simulink model "tx80211a5s"  (R2015b)
settings: Solver=FixedStepDiscrete  SolverMode=SingleTasking  StartTime=0.0  StopTime=46*tpf  RelTol=1e-3
PreLoadFcn:
  | [stx, stb, spi, spq, ntf, cii, cpp, css] = tx80211a_r0;
InitFcn:
  | if ~exist('srx','var')
  | [stx, stb, spi, spq, ntf, cii, cpp, css] = tx80211a_r0;
  | end
  | bitrate = 6e6; % 6 Mbits per second
  | crf = 2; % constant redundancy factor (from conv enc)
  | nepsc = 16; % #empty+pilot subcarriers
  | ncps = 16; % #cyclic prefix samples
  | ndbpf = 24; % #data bits per frame
  | ncbpf = ndbpf * crf; % #coded bits per frame
  | nscpf = ncbpf + nepsc; % #subcarriers per frame
  | nspf = nscpf + 16; % #samples per frame
  | tps = 1e-6; %tpf/nspf; % sample time
  | tpf = tps*nspf; %ndbpf/bitrate; % frame time
values from neighbouring files (symbols this model uses):
  cpp = [1,1,1,1,-1,-1,-1,1,-1,-1,-1,-1,1,1,-1,1,-1,-1,1,1,-1,1,1,-1,1,1,1,1,1,1,-1,1,     1,1,-1,1,1,-1,-1,1,1,1,-1,1,-1,-1,-1,1,-1,1,-1,-1,1,-1,-1,1,1,1,1,1,-1,-1,1,1,     -1,-1,1,-1,1,-1,1,1,-1,-1,-1,1,1,-1,-1,-1,-1,1,-1,-1,1,-1,1,1,1,1,-1,1,-1,1,-1,1,     -1,-1,-1,-1,-1,1,-1,1,1,-1,1,-1,1,1,1,-1,-1,1,-1,-1,-1,1,1,1,-1,-1,-1,-1,-1,-1,-1]    [tx80211a_r0.m]
  css = repmat(logical([0;1;1;0;1;1;0;0;0;0;0;1;1;0;0;1;1;0;1;0;1;0;0;1;1;1;0;0;1;1;1;1;0;1;1;0;1;0;0;0;0;1;0;1;0;1;0;1;1;1;1;1;0;1;0;0;1;0;1;0;0;0;1;1;0;1;1;1;0;0;0;1;1;1;1;1;1;1;0;0;0;0;1;1;1;0;1;1;1;1;0;0;1;0;1;1;0;0;1;0;0;1;0;0;0;0;0;0;1;0;0;0;1;0;0;1;1;0;0;0;1;0;1;1;1;0;1]),2,1)    [tx80211a_r0.m]
  ntf = nzo+1    [tx80211a_r0.m]
  spi = real(spf)    [tx80211a_r0.m]
  spq = imag(spf)    [tx80211a_r0.m]
  stb = [ssb;szb]    [tx80211a_r0.m]
libraries: simulink x41, hdlsllib x35, dspxfrm3 x1, dspsigops x1, commcnvcod2 x1
(part 1 of 2)
settings Model: Creator=wchen  LastModifiedBy=bdroz
settings SolverCC: PositivePriorityOrder=on
settings DataIOCC: SaveFormat=Array  SaveOutput=off  SignalLogging=off  SaveTime=off
settings OptimizationCC: BlockReduction=off  ConditionallyExecuteInputs=off  DefaultParameterBehavior=Inlined  ExpressionDepthLimit=2147483647  OptimizeModelRefInitCode=on  LifeSpan=1  MaxStackSize=64
settings DebuggingCC: AlgebraicLoopMsg=error  UnderspecifiedInitializationDetection=Classic  MergeDetectMultiDrivingBlocksExec=none  SolverPrmCheckMsg=warning  SingleTaskRateTransMsg=error  ParameterPrecisionLossMsg=none  AllowSymbolicDim=on  StateNameClashWarn=warning
settings HardwareCC: ProdBitPerPointer=32  ProdLargestAtomicFloat=None  ProdIntDivRoundTo=Undefined  ProdEndianess=Unspecified  ProdWordSize=32  ProdHWDeviceType=ASIC/FPGA->ASIC/FPGA  TargetBitPerPointer=64  TargetLongLongMode=on  TargetIntDivRoundTo=Zero  TargetEndianess=LittleEndian  TargetWordSize=64  TargetHWDeviceType=MATLAB Host  ProdEqTarget=off
settings RTWCC: SystemTargetFile=ert.tlc  TemplateMakefile=ert_default_tmf  Description=Embedded Coder  GenerateReport=on  Toolchain=Xilinx Software Development Kit (SDK)  IncludeHyperlinkInReport=on  LaunchReport=on  GenerateTraceInfo=on  GenerateTraceReport=on  GenerateTraceReportSl=on  GenerateTraceReportSf=on  GenerateTraceReportEml=on
settings CodeAppCC: ForceParamTrailComments=on  IgnoreCustomStorageClasses=off  OperatorAnnotations=on  SimulinkDataObjDesc=on  SFDataObjDesc=on  MATLABFcnDesc=on  InsertBlockDesc=on  MATLABSourceComments=on
settings ERTTargetCC: ERTCustomFileTemplate=example_file_process.tlc  ConvertIfToSwitch=on  SuppressUnreachableDefaultCases=on
settings ConfigComp: CovModelRefEnable=Off

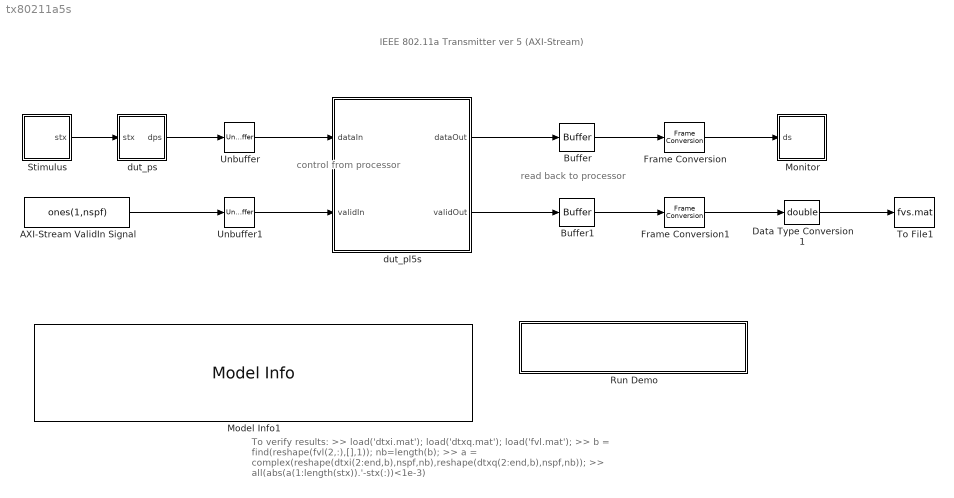
== system tx80211a5s ==
  note: control from
      | processor
  note: IEEE 802.11a Transmitter ver 5 (AXI-Stream)
  note: read back to
      | processor
  note: To verify results:
      | >> load('dtxi.mat'); load('dtxq.mat'); load('fvl.mat');
      | >> b = find(reshape(fvl(2,:),[],1)); nb=length(b);
      | >> a = complex(reshape(dtxi(2:end,b),nspf,nb),reshape(dtxq(2:end,b),nspf,nb));
      | >> all(abs(a(1:length(stx)).'-stx(:))<1e-3)
  AXI-Stream ValidIn Signal : Constant  Value=ones(1,nspf)  OutDataTypeStr=boolean  SampleTime=tpf
  Buffer : Buffer  N=nspf  TreatMby1Signals=One channel  OutputFrames=off
  Buffer1 : Buffer  N=nspf  TreatMby1Signals=One channel  OutputFrames=off
  Data Type Conversion1 : DataTypeConversion  OutDataTypeStr=double
  Frame Conversion : FrameConversion  InheritSamplingMode=off  OutFrame=Sample-based
  Frame Conversion1 : FrameConversion  InheritSamplingMode=off  OutFrame=Sample-based
  Model Info1 : simulink/Model-Wide Utilities/Model Info  Frame=on  DisplayStringWithTags=|  HorizontalTextAlignment=Left  LeftAlignmentValue=0.02  SourceBlockDiagram=tx80211a5s  TagMaxNumber=20
      | This example shows how to use HDL Workflow Advisor to 
      | generate a custom IP core for Zynq SoC evaluation board.
      | 
      | In MATLAB, type the following:
      |   hdladvisor('tx80211a5s/dut_pl5s')
  Monitor : Subsystem
  Run Demo : Subsystem
      settings: OpenFcn=hdladvisor([bdroot, '/led_counter'])
      mask Display: disp('Launch HDL Workflow Advisor')
  Stimulus : Subsystem
  To File1 : ToFile  Filename=fvs.mat  MatrixName=fvs  SampleTime=tpf
  Unbuffer : Unbuffer  SampleBasedProcessing=Same as frame based
  Unbuffer1 : Unbuffer  SampleBasedProcessing=Same as frame based
  dut_pl5s : Subsystem  TreatAsAtomicUnit=on
  dut_ps : Subsystem
  wires:
  Buffer/1 -> Frame Conversion/1
  dut_pl5s/1(dataOut) -> Buffer/1
  Stimulus/1(stx) -> dut_ps/1(stx)
  dut_ps/1(dps) -> Unbuffer/1
  Unbuffer/1 -> dut_pl5s/1(dataIn)
  Frame Conversion/1 -> Monitor/1(ds)
  AXI-Stream ValidIn Signal/1 -> Unbuffer1/1
  Unbuffer1/1 -> dut_pl5s/2(validIn)
  dut_pl5s/2(validOut) -> Buffer1/1
  Buffer1/1 -> Frame Conversion1/1
  Data Type Conversion1/1 -> To File1/1
  Frame Conversion1/1 -> Data Type Conversion1/1

== system tx80211a5s/Monitor ==
  ds : Inport
  Compare To Constant : simulink/Logic and Bit Operations/Compare To Constant  relop=>  const=uint16(0)  OutDataTypeStr=boolean
  Counter Free-Running : simulink/Sources/Counter Free-Running  NumBits=16  tsamp=tpf
  Unpack_int32_into_fix16c1b : Subsystem
  write_srb_to_file : Subsystem
  wires:
  Compare To Constant/1 -> write_srb_to_file/Enable
  Counter Free-Running/1 -> Compare To Constant/1
  ds/1 -> Unpack_int32_into_fix16c1b/1(di32)
  Unpack_int32_into_fix16c1b/2(fvd) -> write_srb_to_file/2(fvl)
  Unpack_int32_into_fix16c1b/1(dts) -> write_srb_to_file/1(srb)

== system tx80211a5s/Run Demo ==

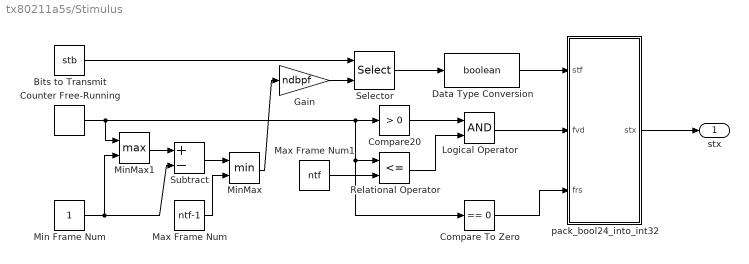
== system tx80211a5s/Stimulus ==
  Bits to Transmit : Constant  Value=stb  SampleTime=tpf
  Compare To Zero : simulink/Logic and Bit Operations/Compare To Zero  relop===  OutDataTypeStr=boolean
  Compare20 : simulink/Logic and Bit Operations/Compare To Zero  relop=>  OutDataTypeStr=boolean
  Counter Free-Running : simulink/Sources/Counter Free-Running  NumBits=16  tsamp=tpf
  Data Type Conversion : DataTypeConversion  OutDataTypeStr=boolean
  Gain : Gain  Gain=ndbpf  OutDataTypeStr=uint16
  Logical Operator : Logic  AllPortsSameDT=off  OutDataTypeStr=boolean
  Max Frame Num : Constant  Value=ntf-1  OutDataTypeStr=uint16  SampleTime=tpf
  Max Frame Num1 : Constant  Value=ntf  OutDataTypeStr=uint16  SampleTime=tpf
  Min Frame Num : Constant  OutDataTypeStr=uint16  SampleTime=tpf
  MinMax : MinMax  Inputs=2  OutDataTypeStr=uint16
  MinMax1 : MinMax  Function=max  Inputs=2
  Relational Operator : RelationalOperator  Operator=<=  OutDataTypeStr=boolean
  Selector : Selector  IndexMode=Zero-based  InputPortWidth=864  IndexOptions=Starting index (port)  Indices=[1 3]  OutputSizes=24
  Subtract : Sum  Inputs=+-  OutDataTypeStr=uint16
  pack_bool24_into_int32 : Subsystem
  stx : Outport
  wires:
  Compare To Zero/1 -> pack_bool24_into_int32/3(frs)
  MinMax1/1 -> Subtract/1
  Subtract/1 -> MinMax/1
  Min Frame Num/1 -> MinMax1/2, Subtract/2
  pack_bool24_into_int32/1(stx) -> stx/1
  Data Type Conversion/1 -> pack_bool24_into_int32/1(stf)
  Selector/1 -> Data Type Conversion/1
  Gain/1 -> Selector/2
  Bits to Transmit/1 -> Selector/1
  MinMax/1 -> Gain/1
  Max Frame Num/1 -> MinMax/2
  Counter Free-Running/1 -> Compare20/1, Relational Operator/1, Compare To Zero/1, MinMax1/1
  Compare20/1 -> Logical Operator/1
  Relational Operator/1 -> Logical Operator/2
  Logical Operator/1 -> pack_bool24_into_int32/2(fvd)
  Max Frame Num1/1 -> Relational Operator/2

== system tx80211a5s/dut_pl5s ==
  dataIn : Inport
  validIn : Inport  Port=2
  PL_dut : Subsystem
  dataOut : Outport  InitialOutput=0
  validOut : Outport  Port=2  InitialOutput=0
  wires:
  dataIn/1 -> PL_dut/1(dps)
  PL_dut/1(dpl) -> dataOut/1
  validIn/1 -> validOut/1, PL_dut/Enable

== system tx80211a5s/dut_ps ==
  stx : Inport
  Logical AND : Logic  IconShape=distinctive  AllPortsSameDT=off  OutDataTypeStr=boolean
  pack_48b_into_int32 : Subsystem
  prepare_frame_ps : Subsystem  TreatAsAtomicUnit=on
  unpack_int32_into_bool24 : Subsystem
  dps : Outport
  wires:
  stx/1 -> unpack_int32_into_bool24/1(di32)
  unpack_int32_into_bool24/3(frs) -> pack_48b_into_int32/3(frs), prepare_frame_ps/2(frs)
  unpack_int32_into_bool24/1(stx) -> prepare_frame_ps/1(stb)
  unpack_int32_into_bool24/2(fvd) -> Logical AND/1, prepare_frame_ps/Enable
  prepare_frame_ps/1(dts) -> pack_48b_into_int32/1(dt48b)
  pack_48b_into_int32/1(dti32) -> dps/1
  Logical AND/1 -> pack_48b_into_int32/2(fvd)
  prepare_frame_ps/2(fvo) -> Logical AND/2

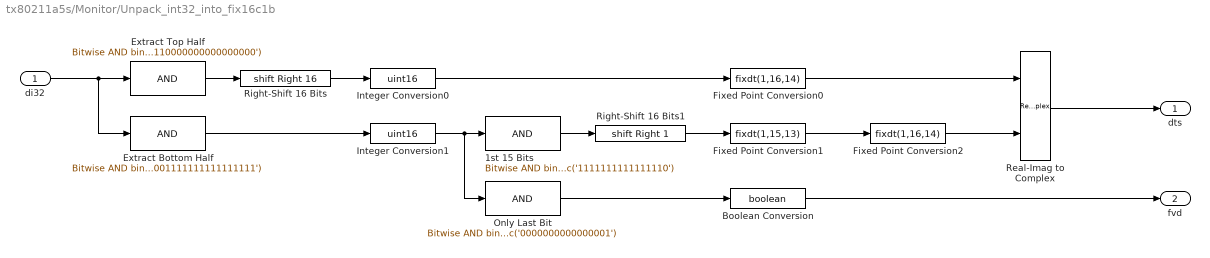
== system tx80211a5s/Monitor/Unpack_int32_into_fix16c1b ==
  di32 : Inport
  1st 15 Bits : simulink/Logic and Bit Operations/Bitwise Operator  logicop=AND  UseBitMask=on  BitMask=bin2dec('1111111111111110')  BitMaskRealWorld=Stored Integer
  Boolean Conversion : DataTypeConversion  OutDataTypeStr=boolean  ConvertRealWorld=Stored Integer (SI)
  Extract Bottom Half : simulink/Logic and Bit Operations/Bitwise Operator  logicop=AND  UseBitMask=on  BitMask=bin2dec('00000000000000001111111111111111')  BitMaskRealWorld=Stored Integer
  Extract Top Half : simulink/Logic and Bit Operations/Bitwise Operator  logicop=AND  UseBitMask=on  BitMask=bin2dec('11111111111111110000000000000000')  BitMaskRealWorld=Stored Integer
  Fixed Point Conversion0 : DataTypeConversion  OutDataTypeStr=fixdt(1,16,14)  ConvertRealWorld=Stored Integer (SI)
      settings: AttributesFormatString=%<OutDataTypeStr>
  Fixed Point Conversion1 : DataTypeConversion  OutDataTypeStr=fixdt(1,15,13)  ConvertRealWorld=Stored Integer (SI)
      settings: AttributesFormatString=%<OutDataTypeStr>
  Fixed Point Conversion2 : DataTypeConversion  OutDataTypeStr=fixdt(1,16,14)
      settings: AttributesFormatString=%<OutDataTypeStr>
  Integer Conversion0 : DataTypeConversion  OutDataTypeStr=uint16  ConvertRealWorld=Stored Integer (SI)
  Integer Conversion1 : DataTypeConversion  OutDataTypeStr=uint16  ConvertRealWorld=Stored Integer (SI)
  Only Last Bit : simulink/Logic and Bit Operations/Bitwise Operator  logicop=AND  UseBitMask=on  BitMask=bin2dec('0000000000000001')  BitMaskRealWorld=Stored Integer
  Real-Imag to Complex : RealImagToComplex
  Right-Shift 16 Bits : ArithShift  BitShiftNumber=16  BitShiftDirection=Right  DiagnosticForOORShift=Error
  Right-Shift 16 Bits1 : ArithShift  BitShiftNumber=1  BitShiftDirection=Right  DiagnosticForOORShift=Error
  dts : Outport
  fvd : Outport  Port=2
  wires:
  Real-Imag to Complex/1 -> dts/1
  Only Last Bit/1 -> Boolean Conversion/1
  Boolean Conversion/1 -> fvd/1
  Fixed Point Conversion0/1 -> Real-Imag to Complex/1
  Fixed Point Conversion2/1 -> Real-Imag to Complex/2
  Extract Bottom Half/1 -> Integer Conversion1/1
  di32/1 -> Extract Bottom Half/1, Extract Top Half/1
  1st 15 Bits/1 -> Right-Shift 16 Bits1/1
  Right-Shift 16 Bits/1 -> Integer Conversion0/1
  Extract Top Half/1 -> Right-Shift 16 Bits/1
  Integer Conversion1/1 -> 1st 15 Bits/1, Only Last Bit/1
  Integer Conversion0/1 -> Fixed Point Conversion0/1
  Fixed Point Conversion1/1 -> Fixed Point Conversion2/1
  Right-Shift 16 Bits1/1 -> Fixed Point Conversion1/1

== system tx80211a5s/Monitor/write_srb_to_file ==
  srb : Inport
  fvl : Inport  Port=2
  Enable : EnablePort
  Complex to Real-Imag : ComplexToRealImag
  Data Type Conversion : DataTypeConversion  OutDataTypeStr=double
  Data Type Conversion1 : DataTypeConversion  OutDataTypeStr=double
  To File : ToFile  Filename=dtxi.mat  MatrixName=dtxi  SampleTime=tpf
  To File1 : ToFile  Filename=fvl.mat  MatrixName=fvl  SampleTime=tpf
  To File2 : ToFile  Filename=dtxq.mat  MatrixName=dtxq  SampleTime=tpf
  wires:
  fvl/1 -> Data Type Conversion1/1
  Data Type Conversion1/1 -> To File1/1
  srb/1 -> Data Type Conversion/1
  Data Type Conversion/1 -> Complex to Real-Imag/1
  Complex to Real-Imag/1 -> To File/1
  Complex to Real-Imag/2 -> To File2/1

== system tx80211a5s/Stimulus/pack_bool24_into_int32 ==
  stf : Inport
  fvd : Inport  Port=2
  frs : Inport  Port=3
  Bit Concat : hdlsllib/HDL Operations/Bit Concat  numInputs=1
  Constant : Constant  Value=false(6,1)  OutDataTypeStr=boolean  SampleTime=tpf
  Vector Concatenate : Concatenate  NumInputs=4
  stx : Outport
  wires:
  Vector Concatenate/1 -> Bit Concat/1
  stf/1 -> Vector Concatenate/1
  fvd/1 -> Vector Concatenate/3
  frs/1 -> Vector Concatenate/4
  Constant/1 -> Vector Concatenate/2
  Bit Concat/1 -> stx/1

== system tx80211a5s/dut_pl5s/PL_dut ==
  dps : Inport
  Enable : EnablePort
  BPSK Modulate : Subsystem  TreatAsAtomicUnit=on
  Interleave : Subsystem  TreatAsAtomicUnit=on
  OFDM Modulate : Subsystem
  Preamble Switch : Subsystem  TreatAsAtomicUnit=on
  Unpack_int32_into_24b : Subsystem
  pack_fpt16c1b_into_int32 : Subsystem
  dpl : Outport  InitialOutput=0
  wires:
  dps/1 -> Unpack_int32_into_24b/1(di32)
  Unpack_int32_into_24b/3(frs) -> Interleave/3(frs), OFDM Modulate/3(frs), Preamble Switch/3(frs)
  OFDM Modulate/2(f8v) -> Preamble Switch/2(f8v)  "f8v"
  pack_fpt16c1b_into_int32/1(dti32) -> dpl/1
  BPSK Modulate/1(s4m) -> OFDM Modulate/1(s4m)
  OFDM Modulate/1(s8s) -> Preamble Switch/1(s8s)
  Preamble Switch/1(s9s) -> pack_fpt16c1b_into_int32/1(dtf16c)
  Preamble Switch/2(f9v) -> pack_fpt16c1b_into_int32/2(fvd)  "f9v"
  BPSK Modulate/2(f4v) -> OFDM Modulate/2(f4v)  "f8v"
  Unpack_int32_into_24b/2(fvd) -> Interleave/2(f3v)  "f8v"
  Unpack_int32_into_24b/1(dts) -> Interleave/1(s2b)
  Interleave/1(s3b) -> BPSK Modulate/1(s3b)
  Interleave/2(f4v) -> BPSK Modulate/2(f3v)

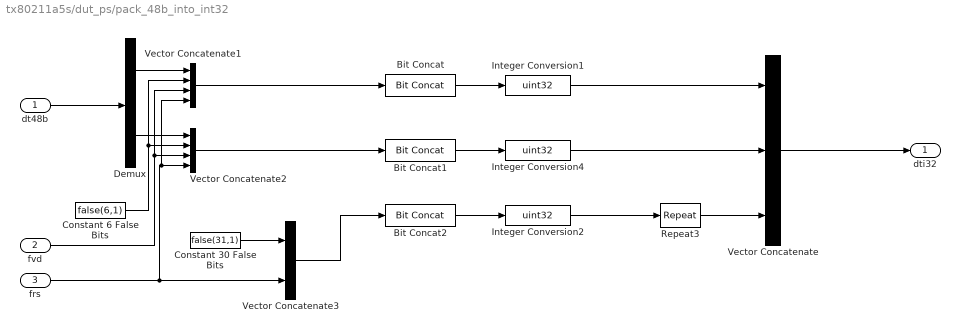
== system tx80211a5s/dut_ps/pack_48b_into_int32 ==
  dt48b : Inport
  fvd : Inport  Port=2
  frs : Inport  Port=3
  Bit Concat : hdlsllib/HDL Operations/Bit Concat  numInputs=1
  Bit Concat1 : hdlsllib/HDL Operations/Bit Concat  numInputs=1
  Bit Concat2 : hdlsllib/HDL Operations/Bit Concat  numInputs=1
  Constant 30 False Bits : Constant  Value=false(31,1)  OutDataTypeStr=boolean  SampleTime=tpf
  Constant 6 False Bits : Constant  Value=false(6,1)  OutDataTypeStr=boolean  SampleTime=tpf
  Demux : Demux  Outputs=2
  Integer Conversion1 : DataTypeConversion  OutDataTypeStr=uint32  ConvertRealWorld=Stored Integer (SI)
  Integer Conversion2 : DataTypeConversion  OutDataTypeStr=uint32  ConvertRealWorld=Stored Integer (SI)
  Integer Conversion4 : DataTypeConversion  OutDataTypeStr=uint32  ConvertRealWorld=Stored Integer (SI)
  Repeat3 : dspsigops/Repeat  N=78  InputProcessing=Columns as channels (frame based)  RateOptions=Enforce single-rate processing  ic=0  mode=Unused parameter value
  Vector Concatenate : Concatenate  NumInputs=3
  Vector Concatenate1 : Concatenate  NumInputs=4
  Vector Concatenate2 : Concatenate  NumInputs=4
  Vector Concatenate3 : Concatenate
  dti32 : Outport
  wires:
  dt48b/1 -> Demux/1
  Vector Concatenate/1 -> dti32/1
  Bit Concat/1 -> Integer Conversion1/1
  Bit Concat1/1 -> Integer Conversion4/1
  Integer Conversion1/1 -> Vector Concatenate/1
  Integer Conversion4/1 -> Vector Concatenate/2
  Demux/1 -> Vector Concatenate1/1
  Demux/2 -> Vector Concatenate2/1
  fvd/1 -> Vector Concatenate1/3, Vector Concatenate2/3
  frs/1 -> Vector Concatenate1/4, Vector Concatenate2/4, Vector Concatenate3/2
  Vector Concatenate1/1 -> Bit Concat/1
  Vector Concatenate2/1 -> Bit Concat1/1
  Constant 6 False Bits/1 -> Vector Concatenate2/2, Vector Concatenate1/2
  Constant 30 False Bits/1 -> Vector Concatenate3/1
  Vector Concatenate3/1 -> Bit Concat2/1
  Bit Concat2/1 -> Integer Conversion2/1
  Integer Conversion2/1 -> Repeat3/1
  Repeat3/1 -> Vector Concatenate/3

== system tx80211a5s/dut_ps/prepare_frame_ps ==
  stb : Inport
  frs : Inport  Port=2
  Enable : EnablePort
  Convolutional Encode : Subsystem  TreatAsAtomicUnit=on
  Scramble : Subsystem  TreatAsAtomicUnit=on
  dts : Outport
  fvo : Outport  Port=2  InitialOutput=0
  wires:
  stb/1 -> Scramble/1(s0b)
  frs/1 -> Scramble/2(frs)
  Scramble/1(s1b) -> Convolutional Encode/1(s1b)
  Scramble/2(f1v) -> Convolutional Encode/2(f1v)
  Convolutional Encode/2(f2v) -> fvo/1
  Convolutional Encode/1(s2b) -> dts/1

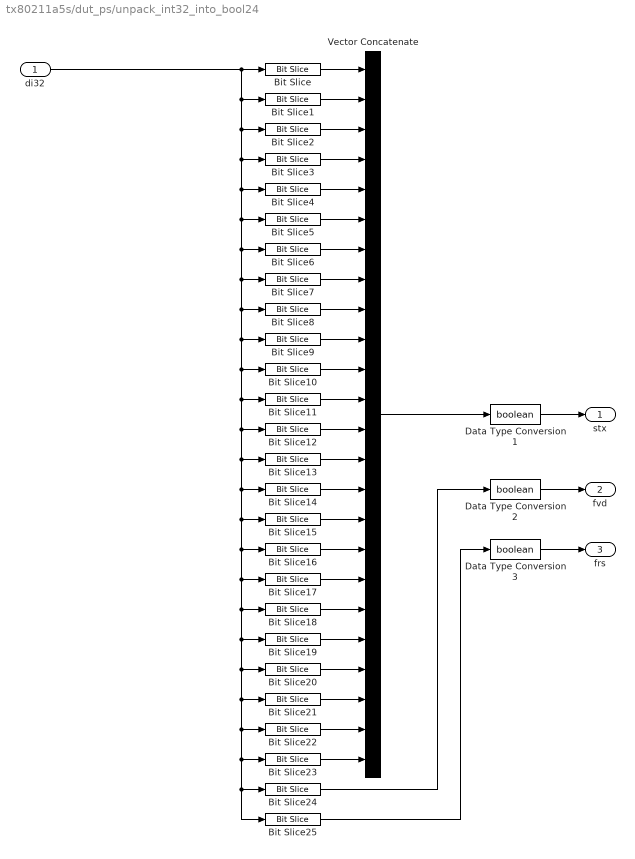
== system tx80211a5s/dut_ps/unpack_int32_into_bool24 ==
  di32 : Inport
  Bit Slice : hdlsllib/HDL Operations/Bit Slice  lidx=31  ridx=31
      settings: AttributesFormatString=%<lidx>
  Bit Slice1 : hdlsllib/HDL Operations/Bit Slice  lidx=30  ridx=30
      settings: AttributesFormatString=%<lidx>
  Bit Slice10 : hdlsllib/HDL Operations/Bit Slice  lidx=21  ridx=21
      settings: AttributesFormatString=%<lidx>
  Bit Slice11 : hdlsllib/HDL Operations/Bit Slice  lidx=20  ridx=20
      settings: AttributesFormatString=%<lidx>
  Bit Slice12 : hdlsllib/HDL Operations/Bit Slice  lidx=19  ridx=19
      settings: AttributesFormatString=%<lidx>
  Bit Slice13 : hdlsllib/HDL Operations/Bit Slice  lidx=18  ridx=18
      settings: AttributesFormatString=%<lidx>
  Bit Slice14 : hdlsllib/HDL Operations/Bit Slice  lidx=17  ridx=17
      settings: AttributesFormatString=%<lidx>
  Bit Slice15 : hdlsllib/HDL Operations/Bit Slice  lidx=16  ridx=16
      settings: AttributesFormatString=%<lidx>
  Bit Slice16 : hdlsllib/HDL Operations/Bit Slice  lidx=15  ridx=15
      settings: AttributesFormatString=%<lidx>
  Bit Slice17 : hdlsllib/HDL Operations/Bit Slice  lidx=14  ridx=14
      settings: AttributesFormatString=%<lidx>
  Bit Slice18 : hdlsllib/HDL Operations/Bit Slice  lidx=13  ridx=13
      settings: AttributesFormatString=%<lidx>
  Bit Slice19 : hdlsllib/HDL Operations/Bit Slice  lidx=12  ridx=12
      settings: AttributesFormatString=%<lidx>
  Bit Slice2 : hdlsllib/HDL Operations/Bit Slice  lidx=29  ridx=29
      settings: AttributesFormatString=%<lidx>
  Bit Slice20 : hdlsllib/HDL Operations/Bit Slice  lidx=11  ridx=11
      settings: AttributesFormatString=%<lidx>
  Bit Slice21 : hdlsllib/HDL Operations/Bit Slice  lidx=10  ridx=10
      settings: AttributesFormatString=%<lidx>
  Bit Slice22 : hdlsllib/HDL Operations/Bit Slice  lidx=9  ridx=9
      settings: AttributesFormatString=%<lidx>
  Bit Slice23 : hdlsllib/HDL Operations/Bit Slice  lidx=8  ridx=8
      settings: AttributesFormatString=%<lidx>
  Bit Slice24 : hdlsllib/HDL Operations/Bit Slice  lidx=1  ridx=1
      settings: AttributesFormatString=%<lidx>
  Bit Slice25 : hdlsllib/HDL Operations/Bit Slice  lidx=0  ridx=0
      settings: AttributesFormatString=%<lidx>
  Bit Slice3 : hdlsllib/HDL Operations/Bit Slice  lidx=28  ridx=28
      settings: AttributesFormatString=%<lidx>
  Bit Slice4 : hdlsllib/HDL Operations/Bit Slice  lidx=27  ridx=27
      settings: AttributesFormatString=%<lidx>
  Bit Slice5 : hdlsllib/HDL Operations/Bit Slice  lidx=26  ridx=26
      settings: AttributesFormatString=%<lidx>
  Bit Slice6 : hdlsllib/HDL Operations/Bit Slice  lidx=25  ridx=25
      settings: AttributesFormatString=%<lidx>
  Bit Slice7 : hdlsllib/HDL Operations/Bit Slice  lidx=24  ridx=24
      settings: AttributesFormatString=%<lidx>
  Bit Slice8 : hdlsllib/HDL Operations/Bit Slice  lidx=23  ridx=23
      settings: AttributesFormatString=%<lidx>
  Bit Slice9 : hdlsllib/HDL Operations/Bit Slice  lidx=22  ridx=22
      settings: AttributesFormatString=%<lidx>
  Data Type Conversion1 : DataTypeConversion  OutDataTypeStr=boolean
  Data Type Conversion2 : DataTypeConversion  OutDataTypeStr=boolean
  Data Type Conversion3 : DataTypeConversion  OutDataTypeStr=boolean
  Vector Concatenate : Concatenate  NumInputs=24
  stx : Outport
  fvd : Outport  Port=2
  frs : Outport  Port=3
  wires:
  Vector Concatenate/1 -> Data Type Conversion1/1
  Bit Slice25/1 -> Data Type Conversion3/1
  Bit Slice24/1 -> Data Type Conversion2/1
  di32/1 -> Bit Slice1/1, Bit Slice2/1, Bit Slice3/1, Bit Slice4/1, Bit Slice5/1, Bit Slice7/1, Bit Slice8/1, Bit Slice9/1, Bit Slice11/1, Bit Slice12/1, Bit Slice13/1, Bit Slice15/1, Bit Slice17/1, Bit Slice18/1, Bit Slice19/1, Bit Slice20/1, Bit Slice21/1, Bit Slice25/1, Bit Slice24/1, Bit Slice23/1, Bit Slice22/1, Bit Slice16/1, Bit Slice14/1, Bit Slice10/1, Bit Slice6/1, Bit Slice/1
  Bit Slice23/1 -> Vector Concatenate/24
  Bit Slice22/1 -> Vector Concatenate/23
  Bit Slice21/1 -> Vector Concatenate/22
  Bit Slice20/1 -> Vector Concatenate/21
  Bit Slice19/1 -> Vector Concatenate/20
  Bit Slice18/1 -> Vector Concatenate/19
  Bit Slice17/1 -> Vector Concatenate/18
  Bit Slice16/1 -> Vector Concatenate/17
  Bit Slice15/1 -> Vector Concatenate/16
  Bit Slice14/1 -> Vector Concatenate/15
  Bit Slice13/1 -> Vector Concatenate/14
  Bit Slice12/1 -> Vector Concatenate/13
  Bit Slice11/1 -> Vector Concatenate/12
  Bit Slice10/1 -> Vector Concatenate/11
  Bit Slice9/1 -> Vector Concatenate/10
  Bit Slice8/1 -> Vector Concatenate/9
  Bit Slice7/1 -> Vector Concatenate/8
  Bit Slice6/1 -> Vector Concatenate/7
  Bit Slice5/1 -> Vector Concatenate/6
  Bit Slice4/1 -> Vector Concatenate/5
  Bit Slice3/1 -> Vector Concatenate/4
  Bit Slice2/1 -> Vector Concatenate/3
  Bit Slice1/1 -> Vector Concatenate/2
  Bit Slice/1 -> Vector Concatenate/1
  Data Type Conversion1/1 -> stx/1
  Data Type Conversion2/1 -> fvd/1
  Data Type Conversion3/1 -> frs/1

== system tx80211a5s/dut_pl5s/PL_dut/BPSK Modulate ==
  s3b : Inport
  f3v : Inport  Port=2
  BPSK Modulate Baseband : Subsystem
  s4m : Outport
  f4v : Outport  Port=2
  wires:
  f3v/1 -> f4v/1
  s3b/1 -> BPSK Modulate Baseband/1(bits)
  BPSK Modulate Baseband/1(symbols) -> s4m/1

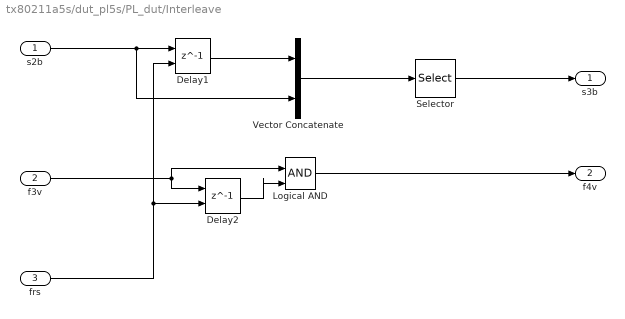
== system tx80211a5s/dut_pl5s/PL_dut/Interleave ==
  s2b : Inport
  f3v : Inport  Port=2
  frs : Inport  Port=3
  Delay1 : Delay  DelayLength=1  ExternalReset=Level  SampleTime=tps
      settings: InputPortMap=u0,r5
  Delay2 : Delay  DelayLength=1  ExternalReset=Level  SampleTime=tps
      settings: InputPortMap=u0,r5
  Logical AND : Logic  IconShape=distinctive  AllPortsSameDT=off  OutDataTypeStr=boolean
  Selector : Selector  IndexMode=Zero-based  InputPortWidth=48  IndexOptions=Index vector (dialog)  Indices=cii  OutputSizes=1
  Vector Concatenate : Concatenate
  s3b : Outport
  f4v : Outport  Port=2
  wires:
  f3v/1 -> Logical AND/1, Delay2/1
  frs/1 -> Delay2/2, Delay1/2
  Delay2/1 -> Logical AND/2
  Logical AND/1 -> f4v/1
  Vector Concatenate/1 -> Selector/1
  Delay1/1 -> Vector Concatenate/1
  s2b/1 -> Vector Concatenate/2, Delay1/1
  Selector/1 -> s3b/1

== system tx80211a5s/dut_pl5s/PL_dut/OFDM Modulate ==
  s4m : Inport
  f4v : Inport  Port=2
  frs : Inport  Port=3
  Frame-Based to Sample-Based : Subsystem
  IFFT HDL Optimized : dspxfrm3/IFFT HDL Optimized  BitReversedOutput=off  Normalize=on  FFTLengthSource=Property  FFTLength=64  RoundingMethod=Floor  OverflowAction=Saturate  ValidInputPort=on  ResetInputPort=on  StartOutputPort=off  EndOutputPort=off  SimulateUsing=Code generation
  Map Symbols to Subcarriers : Subsystem
  Prepend Cyclic Prefix : Subsystem  TreatAsAtomicUnit=on
  s8s : Outport
  f8v : Outport  Port=2
  wires:
  Prepend Cyclic Prefix/1(s8s) -> s8s/1
  Prepend Cyclic Prefix/2(f8v) -> f8v/1  "f8v"
  frs/1 -> Frame-Based to Sample-Based/3(frs), IFFT HDL Optimized/3, Prepend Cyclic Prefix/3(frs), Map Symbols to Subcarriers/3(frs)
  Map Symbols to Subcarriers/2(f5v) -> Frame-Based to Sample-Based/2(f5v)  "f5v"
  s4m/1 -> Map Symbols to Subcarriers/1(s4m)
  f4v/1 -> Map Symbols to Subcarriers/2(f4v)  "f4v"
  Map Symbols to Subcarriers/1(s5m) -> Frame-Based to Sample-Based/1(s5m)
  Frame-Based to Sample-Based/2(f6v) -> IFFT HDL Optimized/2  "f5v"
  Frame-Based to Sample-Based/1(s6m) -> IFFT HDL Optimized/1
  IFFT HDL Optimized/2 -> Prepend Cyclic Prefix/2(f7v)  "f5v"
  IFFT HDL Optimized/1 -> Prepend Cyclic Prefix/1(s7s)

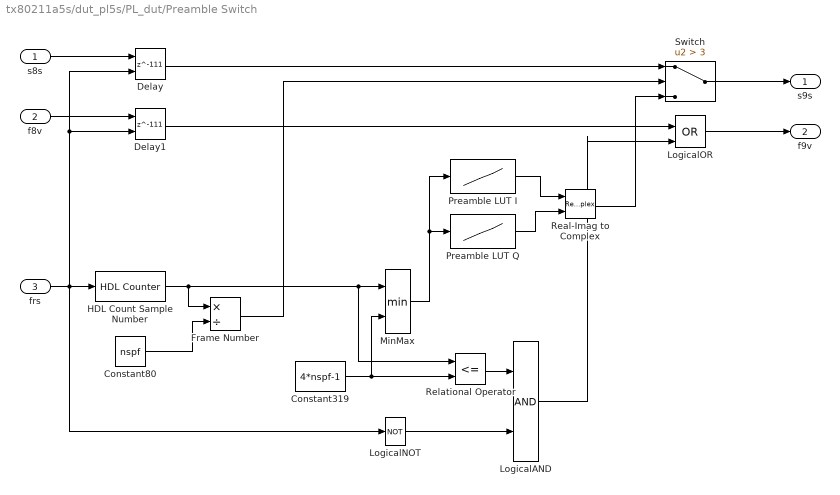
== system tx80211a5s/dut_pl5s/PL_dut/Preamble Switch ==
  s8s : Inport
  f8v : Inport  Port=2
  frs : Inport  Port=3
  Constant319 : Constant  Value=4*nspf-1  OutDataTypeStr=uint16  SampleTime=tps
  Constant80 : Constant  Value=nspf  OutDataTypeStr=uint8  SampleTime=tps
  Delay : Delay  DelayLength=111  ExternalReset=Level  SampleTime=tps
      settings: InputPortMap=u0,r5
  Delay1 : Delay  DelayLength=111  InitialCondition=false  ExternalReset=Level  SampleTime=tps
      settings: InputPortMap=u0,r5
  Frame Number : Product  Inputs=*/  OutDataTypeStr=uint16  SaturateOnIntegerOverflow=on  RndMeth=Zero
  HDL Count Sample Number : hdlsllib/HDL Operations/HDL Counter  CountType=Free running  CountInit=0  CountStep=1  CountMax=3  CountFromType=Initial value  CountFrom=0  CountResetPort=on  CountLoadPort=off  CountEnbPort=off  CountDirPort=off  CountDataType=Unsigned  CountWordLen=16  CountFracLen=0  CountSampTime=1
  LogicalAND : Logic  IconShape=distinctive  AllPortsSameDT=off  OutDataTypeStr=boolean
  LogicalNOT : Logic  Operator=NOT  IconShape=distinctive  AllPortsSameDT=off  OutDataTypeStr=boolean
  LogicalOR : Logic  Operator=OR  IconShape=distinctive  AllPortsSameDT=off  OutDataTypeStr=boolean
  MinMax : MinMax  Inputs=2
  Preamble LUT I : Lookup_n-D  NumberOfTableDimensions=1  BreakpointsForDimension1=[0:1:319]  BreakpointsForDimension1FirstPoint=10  BreakpointsForDimension2FirstPoint=10  BreakpointsForDimension1Spacing=12  BreakpointsForDimension2Spacing=12  IndexSearchMethod=Evenly spaced points  Table=spi  InterpMethod=Flat  DiagnosticForOutOfRangeInput=Error  InternalRulePriority=Speed  OutDataTypeStr=fixdt(1,16,14)  RndMeth=Simplest  InputSameDT=on
  Preamble LUT Q : Lookup_n-D  NumberOfTableDimensions=1  BreakpointsForDimension1=[0:1:319]  BreakpointsForDimension1FirstPoint=10  BreakpointsForDimension2FirstPoint=10  BreakpointsForDimension1Spacing=12  BreakpointsForDimension2Spacing=12  IndexSearchMethod=Evenly spaced points  Table=spq  TableDataTypeStr=fixdt(1,16,14)  InterpMethod=Flat  DiagnosticForOutOfRangeInput=Error  InternalRulePriority=Speed  OutDataTypeStr=fixdt(1,16,14)  RndMeth=Simplest  InputSameDT=on
  Real-Imag to Complex : RealImagToComplex
  Relational Operator : RelationalOperator  Operator=<=  OutDataTypeStr=boolean
  Switch : Switch  Criteria=u2 > Threshold  Threshold=3
  s9s : Outport
  f9v : Outport  Port=2
  wires:
  f8v/1 -> Delay1/1
  frs/1 -> Delay/2, Delay1/2, LogicalNOT/1, HDL Count Sample Number/1
  Switch/1 -> s9s/1
  s8s/1 -> Delay/1
  Real-Imag to Complex/1 -> Switch/3
  Constant80/1 -> Frame Number/2
  Delay/1 -> Switch/1
  Frame Number/1 -> Switch/2
  HDL Count Sample Number/1 -> Relational Operator/1, MinMax/1, Frame Number/1
  Constant319/1 -> MinMax/2, Relational Operator/2
  MinMax/1 -> Preamble LUT Q/1, Preamble LUT I/1
  LogicalOR/1 -> f9v/1
  LogicalNOT/1 -> LogicalAND/2
  Relational Operator/1 -> LogicalAND/1
  LogicalAND/1 -> LogicalOR/2
  Delay1/1 -> LogicalOR/1
  Preamble LUT I/1 -> Real-Imag to Complex/1
  Preamble LUT Q/1 -> Real-Imag to Complex/2

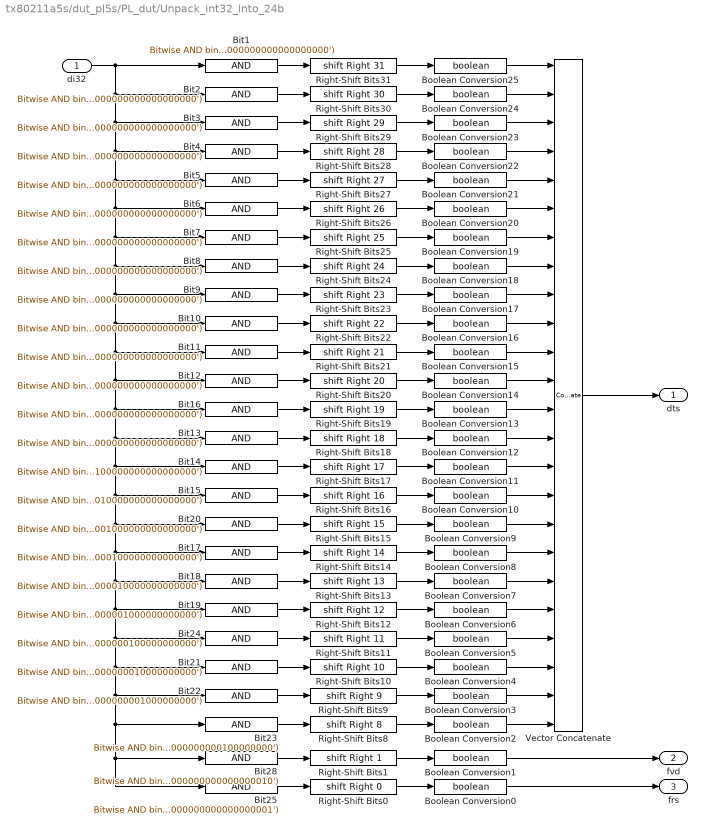
== system tx80211a5s/dut_pl5s/PL_dut/Unpack_int32_into_24b ==
  di32 : Inport
  Bit1 : simulink/Logic and Bit Operations/Bitwise Operator  logicop=AND  UseBitMask=on  BitMask=bin2dec('10000000000000000000000000000000')  BitMaskRealWorld=Stored Integer
      settings: AttributesFormatString=%<logicop>%<BitMask>
  Bit10 : simulink/Logic and Bit Operations/Bitwise Operator  logicop=AND  UseBitMask=on  BitMask=bin2dec('00000000010000000000000000000000')  BitMaskRealWorld=Stored Integer
      settings: AttributesFormatString=%<logicop>%<BitMask>
  Bit11 : simulink/Logic and Bit Operations/Bitwise Operator  logicop=AND  UseBitMask=on  BitMask=bin2dec('00000000001000000000000000000000')  BitMaskRealWorld=Stored Integer
      settings: AttributesFormatString=%<logicop>%<BitMask>
  Bit12 : simulink/Logic and Bit Operations/Bitwise Operator  logicop=AND  UseBitMask=on  BitMask=bin2dec('00000000000100000000000000000000')  BitMaskRealWorld=Stored Integer
      settings: AttributesFormatString=%<logicop>%<BitMask>
  Bit13 : simulink/Logic and Bit Operations/Bitwise Operator  logicop=AND  UseBitMask=on  BitMask=bin2dec('00000000000001000000000000000000')  BitMaskRealWorld=Stored Integer
      settings: AttributesFormatString=%<logicop>%<BitMask>
  Bit14 : simulink/Logic and Bit Operations/Bitwise Operator  logicop=AND  UseBitMask=on  BitMask=bin2dec('00000000000000100000000000000000')  BitMaskRealWorld=Stored Integer
      settings: AttributesFormatString=%<logicop>%<BitMask>
  Bit15 : simulink/Logic and Bit Operations/Bitwise Operator  logicop=AND  UseBitMask=on  BitMask=bin2dec('00000000000000010000000000000000')  BitMaskRealWorld=Stored Integer
      settings: AttributesFormatString=%<logicop>%<BitMask>
  Bit16 : simulink/Logic and Bit Operations/Bitwise Operator  logicop=AND  UseBitMask=on  BitMask=bin2dec('00000000000010000000000000000000')  BitMaskRealWorld=Stored Integer
      settings: AttributesFormatString=%<logicop>%<BitMask>
  Bit17 : simulink/Logic and Bit Operations/Bitwise Operator  logicop=AND  UseBitMask=on  BitMask=bin2dec('00000000000000000100000000000000')  BitMaskRealWorld=Stored Integer
      settings: AttributesFormatString=%<logicop>%<BitMask>
  Bit18 : simulink/Logic and Bit Operations/Bitwise Operator  logicop=AND  UseBitMask=on  BitMask=bin2dec('00000000000000000010000000000000')  BitMaskRealWorld=Stored Integer
      settings: AttributesFormatString=%<logicop>%<BitMask>
  Bit19 : simulink/Logic and Bit Operations/Bitwise Operator  logicop=AND  UseBitMask=on  BitMask=bin2dec('00000000000000000001000000000000')  BitMaskRealWorld=Stored Integer
      settings: AttributesFormatString=%<logicop>%<BitMask>
  Bit2 : simulink/Logic and Bit Operations/Bitwise Operator  logicop=AND  UseBitMask=on  BitMask=bin2dec('01000000000000000000000000000000')  BitMaskRealWorld=Stored Integer
      settings: AttributesFormatString=%<logicop>%<BitMask>
  Bit20 : simulink/Logic and Bit Operations/Bitwise Operator  logicop=AND  UseBitMask=on  BitMask=bin2dec('00000000000000001000000000000000')  BitMaskRealWorld=Stored Integer
      settings: AttributesFormatString=%<logicop>%<BitMask>
  Bit21 : simulink/Logic and Bit Operations/Bitwise Operator  logicop=AND  UseBitMask=on  BitMask=bin2dec('00000000000000000000010000000000')  BitMaskRealWorld=Stored Integer
      settings: AttributesFormatString=%<logicop>%<BitMask>
  Bit22 : simulink/Logic and Bit Operations/Bitwise Operator  logicop=AND  UseBitMask=on  BitMask=bin2dec('00000000000000000000001000000000')  BitMaskRealWorld=Stored Integer
      settings: AttributesFormatString=%<logicop>%<BitMask>
  Bit23 : simulink/Logic and Bit Operations/Bitwise Operator  logicop=AND  UseBitMask=on  BitMask=bin2dec('00000000000000000000000100000000')  BitMaskRealWorld=Stored Integer
      settings: AttributesFormatString=%<logicop>%<BitMask>
  Bit24 : simulink/Logic and Bit Operations/Bitwise Operator  logicop=AND  UseBitMask=on  BitMask=bin2dec('00000000000000000000100000000000')  BitMaskRealWorld=Stored Integer
      settings: AttributesFormatString=%<logicop>%<BitMask>
  Bit25 : simulink/Logic and Bit Operations/Bitwise Operator  logicop=AND  UseBitMask=on  BitMask=bin2dec('00000000000000000000000000000001')  BitMaskRealWorld=Stored Integer
      settings: AttributesFormatString=%<logicop>%<BitMask>
  Bit28 : simulink/Logic and Bit Operations/Bitwise Operator  logicop=AND  UseBitMask=on  BitMask=bin2dec('00000000000000000000000000000010')  BitMaskRealWorld=Stored Integer
      settings: AttributesFormatString=%<logicop>%<BitMask>
  Bit3 : simulink/Logic and Bit Operations/Bitwise Operator  logicop=AND  UseBitMask=on  BitMask=bin2dec('00100000000000000000000000000000')  BitMaskRealWorld=Stored Integer
      settings: AttributesFormatString=%<logicop>%<BitMask>
  Bit4 : simulink/Logic and Bit Operations/Bitwise Operator  logicop=AND  UseBitMask=on  BitMask=bin2dec('00010000000000000000000000000000')  BitMaskRealWorld=Stored Integer
      settings: AttributesFormatString=%<logicop>%<BitMask>
  Bit5 : simulink/Logic and Bit Operations/Bitwise Operator  logicop=AND  UseBitMask=on  BitMask=bin2dec('00001000000000000000000000000000')  BitMaskRealWorld=Stored Integer
      settings: AttributesFormatString=%<logicop>%<BitMask>
  Bit6 : simulink/Logic and Bit Operations/Bitwise Operator  logicop=AND  UseBitMask=on  BitMask=bin2dec('00000100000000000000000000000000')  BitMaskRealWorld=Stored Integer
      settings: AttributesFormatString=%<logicop>%<BitMask>
  Bit7 : simulink/Logic and Bit Operations/Bitwise Operator  logicop=AND  UseBitMask=on  BitMask=bin2dec('00000010000000000000000000000000')  BitMaskRealWorld=Stored Integer
      settings: AttributesFormatString=%<logicop>%<BitMask>
  Bit8 : simulink/Logic and Bit Operations/Bitwise Operator  logicop=AND  UseBitMask=on  BitMask=bin2dec('00000001000000000000000000000000')  BitMaskRealWorld=Stored Integer
      settings: AttributesFormatString=%<logicop>%<BitMask>
  Bit9 : simulink/Logic and Bit Operations/Bitwise Operator  logicop=AND  UseBitMask=on  BitMask=bin2dec('00000000100000000000000000000000')  BitMaskRealWorld=Stored Integer
      settings: AttributesFormatString=%<logicop>%<BitMask>
  Boolean Conversion{0..25} (26 alike) : DataTypeConversion  OutDataTypeStr=boolean  ConvertRealWorld=Stored Integer (SI)
  Right-Shift Bits0 : ArithShift  BitShiftDirection=Right  DiagnosticForOORShift=Error
  Right-Shift Bits1 : ArithShift  BitShiftNumber=1  BitShiftDirection=Right  DiagnosticForOORShift=Error
  Right-Shift Bits10 : ArithShift  BitShiftNumber=10  BitShiftDirection=Right  DiagnosticForOORShift=Error
  Right-Shift Bits11 : ArithShift  BitShiftNumber=11  BitShiftDirection=Right  DiagnosticForOORShift=Error
  Right-Shift Bits12 : ArithShift  BitShiftNumber=12  BitShiftDirection=Right  DiagnosticForOORShift=Error
  Right-Shift Bits13 : ArithShift  BitShiftNumber=13  BitShiftDirection=Right  DiagnosticForOORShift=Error
  Right-Shift Bits14 : ArithShift  BitShiftNumber=14  BitShiftDirection=Right  DiagnosticForOORShift=Error
  Right-Shift Bits15 : ArithShift  BitShiftNumber=15  BitShiftDirection=Right  DiagnosticForOORShift=Error
  Right-Shift Bits16 : ArithShift  BitShiftNumber=16  BitShiftDirection=Right  DiagnosticForOORShift=Error
  Right-Shift Bits17 : ArithShift  BitShiftNumber=17  BitShiftDirection=Right  DiagnosticForOORShift=Error
  Right-Shift Bits18 : ArithShift  BitShiftNumber=18  BitShiftDirection=Right  DiagnosticForOORShift=Error
  Right-Shift Bits19 : ArithShift  BitShiftNumber=19  BitShiftDirection=Right  DiagnosticForOORShift=Error
  Right-Shift Bits20 : ArithShift  BitShiftNumber=20  BitShiftDirection=Right  DiagnosticForOORShift=Error
  Right-Shift Bits21 : ArithShift  BitShiftNumber=21  BitShiftDirection=Right  DiagnosticForOORShift=Error
  Right-Shift Bits22 : ArithShift  BitShiftNumber=22  BitShiftDirection=Right  DiagnosticForOORShift=Error
  Right-Shift Bits23 : ArithShift  BitShiftNumber=23  BitShiftDirection=Right  DiagnosticForOORShift=Error
  Right-Shift Bits24 : ArithShift  BitShiftNumber=24  BitShiftDirection=Right  DiagnosticForOORShift=Error
  Right-Shift Bits25 : ArithShift  BitShiftNumber=25  BitShiftDirection=Right  DiagnosticForOORShift=Error
  Right-Shift Bits26 : ArithShift  BitShiftNumber=26  BitShiftDirection=Right  DiagnosticForOORShift=Error
  Right-Shift Bits27 : ArithShift  BitShiftNumber=27  BitShiftDirection=Right  DiagnosticForOORShift=Error
  Right-Shift Bits28 : ArithShift  BitShiftNumber=28  BitShiftDirection=Right  DiagnosticForOORShift=Error
  Right-Shift Bits29 : ArithShift  BitShiftNumber=29  BitShiftDirection=Right  DiagnosticForOORShift=Error
  Right-Shift Bits30 : ArithShift  BitShiftNumber=30  BitShiftDirection=Right  DiagnosticForOORShift=Error
  Right-Shift Bits31 : ArithShift  BitShiftNumber=31  BitShiftDirection=Right  DiagnosticForOORShift=Error
  Right-Shift Bits8 : ArithShift  BitShiftNumber=8  BitShiftDirection=Right  DiagnosticForOORShift=Error
  Right-Shift Bits9 : ArithShift  BitShiftNumber=9  BitShiftDirection=Right  DiagnosticForOORShift=Error
  Vector Concatenate : Concatenate  NumInputs=24
  dts : Outport
  fvd : Outport  Port=2
  frs : Outport  Port=3
  wires:
  Vector Concatenate/1 -> dts/1
  di32/1 -> Bit2/1, Bit4/1, Bit5/1, Bit6/1, Bit7/1, Bit8/1, Bit9/1, Bit10/1, Bit12/1, Bit16/1, Bit13/1, Bit14/1, Bit15/1, Bit20/1, Bit17/1, Bit18/1, Bit19/1, Bit24/1, Bit21/1, Bit22/1, Bit23/1, Bit28/1, Bit25/1, Bit11/1, Bit3/1, Bit1/1
  Bit1/1 -> Right-Shift Bits31/1
  Bit2/1 -> Right-Shift Bits30/1
  Bit3/1 -> Right-Shift Bits29/1
  Bit4/1 -> Right-Shift Bits28/1
  Bit5/1 -> Right-Shift Bits27/1
  Bit6/1 -> Right-Shift Bits26/1
  Bit7/1 -> Right-Shift Bits25/1
  Bit8/1 -> Right-Shift Bits24/1
  Bit9/1 -> Right-Shift Bits23/1
  Bit10/1 -> Right-Shift Bits22/1
  Bit11/1 -> Right-Shift Bits21/1
  Bit12/1 -> Right-Shift Bits20/1
  Bit16/1 -> Right-Shift Bits19/1
  Bit13/1 -> Right-Shift Bits18/1
  Bit14/1 -> Right-Shift Bits17/1
  Bit15/1 -> Right-Shift Bits16/1
  Bit20/1 -> Right-Shift Bits15/1
  Bit17/1 -> Right-Shift Bits14/1
  Bit18/1 -> Right-Shift Bits13/1
  Bit19/1 -> Right-Shift Bits12/1
  Bit24/1 -> Right-Shift Bits11/1
  Bit21/1 -> Right-Shift Bits10/1
  Bit22/1 -> Right-Shift Bits9/1
  Bit23/1 -> Right-Shift Bits8/1
  Bit28/1 -> Right-Shift Bits1/1
  Bit25/1 -> Right-Shift Bits0/1
  Right-Shift Bits31/1 -> Boolean Conversion25/1
  Right-Shift Bits30/1 -> Boolean Conversion24/1
  Right-Shift Bits29/1 -> Boolean Conversion23/1
  Right-Shift Bits28/1 -> Boolean Conversion22/1
  Right-Shift Bits27/1 -> Boolean Conversion21/1
  Right-Shift Bits26/1 -> Boolean Conversion20/1
  Right-Shift Bits25/1 -> Boolean Conversion19/1
  Right-Shift Bits24/1 -> Boolean Conversion18/1
  Right-Shift Bits23/1 -> Boolean Conversion17/1
  Right-Shift Bits22/1 -> Boolean Conversion16/1
  Right-Shift Bits21/1 -> Boolean Conversion15/1
  Right-Shift Bits20/1 -> Boolean Conversion14/1
  Right-Shift Bits19/1 -> Boolean Conversion13/1
  Right-Shift Bits18/1 -> Boolean Conversion12/1
  Right-Shift Bits17/1 -> Boolean Conversion11/1
  Right-Shift Bits16/1 -> Boolean Conversion10/1
  Right-Shift Bits15/1 -> Boolean Conversion9/1
  Right-Shift Bits14/1 -> Boolean Conversion8/1
  Right-Shift Bits13/1 -> Boolean Conversion7/1
  Right-Shift Bits12/1 -> Boolean Conversion6/1
  Right-Shift Bits11/1 -> Boolean Conversion5/1
  Right-Shift Bits10/1 -> Boolean Conversion4/1
  Right-Shift Bits9/1 -> Boolean Conversion3/1
  Right-Shift Bits8/1 -> Boolean Conversion2/1
  Right-Shift Bits1/1 -> Boolean Conversion1/1
  Right-Shift Bits0/1 -> Boolean Conversion0/1
  Boolean Conversion25/1 -> Vector Concatenate/1
  Boolean Conversion24/1 -> Vector Concatenate/2
  Boolean Conversion23/1 -> Vector Concatenate/3
  Boolean Conversion22/1 -> Vector Concatenate/4
  Boolean Conversion21/1 -> Vector Concatenate/5
  Boolean Conversion20/1 -> Vector Concatenate/6
  Boolean Conversion19/1 -> Vector Concatenate/7
  Boolean Conversion18/1 -> Vector Concatenate/8
  Boolean Conversion17/1 -> Vector Concatenate/9
  Boolean Conversion16/1 -> Vector Concatenate/10
  Boolean Conversion15/1 -> Vector Concatenate/11
  Boolean Conversion14/1 -> Vector Concatenate/12
  Boolean Conversion13/1 -> Vector Concatenate/13
  Boolean Conversion12/1 -> Vector Concatenate/14
  Boolean Conversion11/1 -> Vector Concatenate/15
  Boolean Conversion10/1 -> Vector Concatenate/16
  Boolean Conversion9/1 -> Vector Concatenate/17
  Boolean Conversion8/1 -> Vector Concatenate/18
  Boolean Conversion7/1 -> Vector Concatenate/19
  Boolean Conversion6/1 -> Vector Concatenate/20
  Boolean Conversion5/1 -> Vector Concatenate/21
  Boolean Conversion4/1 -> Vector Concatenate/22
  Boolean Conversion3/1 -> Vector Concatenate/23
  Boolean Conversion2/1 -> Vector Concatenate/24
  Boolean Conversion1/1 -> fvd/1
  Boolean Conversion0/1 -> frs/1

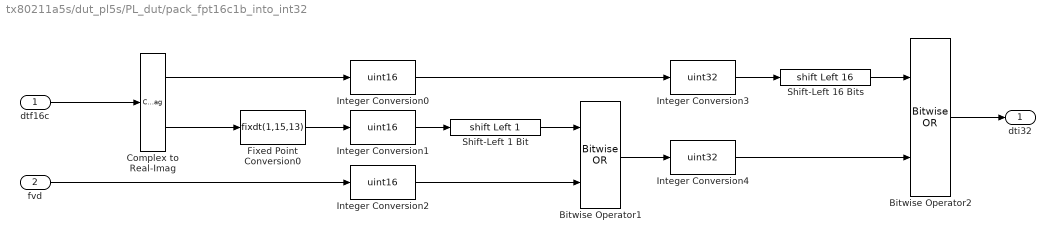
== system tx80211a5s/dut_pl5s/PL_dut/pack_fpt16c1b_into_int32 ==
  dtf16c : Inport
  fvd : Inport  Port=2
  Bitwise Operator1 : simulink/Logic and Bit Operations/Bitwise Operator  logicop=OR  UseBitMask=off  NumInputPorts=2  BitMask=bin2dec('11011001')  BitMaskRealWorld=Stored Integer
  Bitwise Operator2 : simulink/Logic and Bit Operations/Bitwise Operator  logicop=OR  UseBitMask=off  NumInputPorts=2  BitMask=bin2dec('11011001')  BitMaskRealWorld=Stored Integer
  Complex to Real-Imag : ComplexToRealImag
  Fixed Point Conversion0 : DataTypeConversion  OutDataTypeStr=fixdt(1,15,13)
      settings: AttributesFormatString=%<OutDataTypeStr>
  Integer Conversion0 : DataTypeConversion  OutDataTypeStr=uint16  ConvertRealWorld=Stored Integer (SI)
  Integer Conversion1 : DataTypeConversion  OutDataTypeStr=uint16  ConvertRealWorld=Stored Integer (SI)
  Integer Conversion2 : DataTypeConversion  OutDataTypeStr=uint16  ConvertRealWorld=Stored Integer (SI)
  Integer Conversion3 : DataTypeConversion  OutDataTypeStr=uint32  ConvertRealWorld=Stored Integer (SI)
  Integer Conversion4 : DataTypeConversion  OutDataTypeStr=uint32  ConvertRealWorld=Stored Integer (SI)
  Shift-Left 1 Bit : ArithShift  BitShiftNumber=1  BitShiftDirection=Left  DiagnosticForOORShift=Error
  Shift-Left 16 Bits : ArithShift  BitShiftNumber=16  BitShiftDirection=Left  DiagnosticForOORShift=Error
  dti32 : Outport
  wires:
  Bitwise Operator2/1 -> dti32/1
  dtf16c/1 -> Complex to Real-Imag/1
  Complex to Real-Imag/2 -> Fixed Point Conversion0/1
  fvd/1 -> Integer Conversion2/1
  Integer Conversion2/1 -> Bitwise Operator1/2
  Integer Conversion1/1 -> Shift-Left 1 Bit/1
  Bitwise Operator1/1 -> Integer Conversion4/1
  Complex to Real-Imag/1 -> Integer Conversion0/1
  Integer Conversion0/1 -> Integer Conversion3/1
  Integer Conversion3/1 -> Shift-Left 16 Bits/1
  Shift-Left 16 Bits/1 -> Bitwise Operator2/1
  Integer Conversion4/1 -> Bitwise Operator2/2
  Fixed Point Conversion0/1 -> Integer Conversion1/1
  Shift-Left 1 Bit/1 -> Bitwise Operator1/1

== system tx80211a5s/dut_ps/prepare_frame_ps/Convolutional Encode ==
  s1b : Inport
  f1v : Inport  Port=2
  Convolutional Encoder : commcnvcod2/Convolutional Encoder  trellis=poly2trellis(7, [133,171])  opMode=Continuous  DelayedResetAction=on  hasIniStPort=off  hasFinStPort=off  usePuncVector=off  punctureVector=[1; 1; 0; 1; 0; 1]  reset=Unused parameter value
  s2b : Outport
  f2v : Outport  Port=2
  wires:
  f1v/1 -> f2v/1
  s1b/1 -> Convolutional Encoder/1
  Convolutional Encoder/1 -> s2b/1

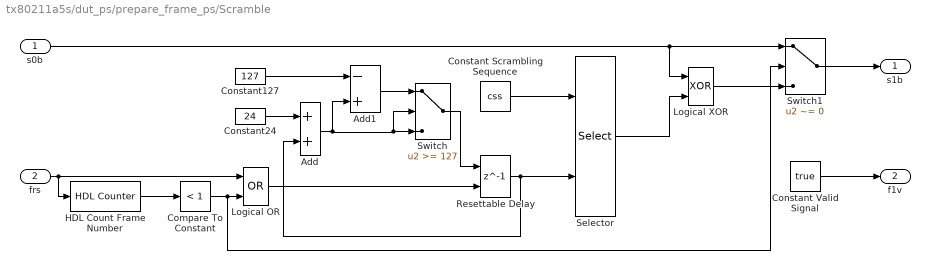
== system tx80211a5s/dut_ps/prepare_frame_ps/Scramble ==
  s0b : Inport
  frs : Inport  Port=2
  Add : Sum  AccumDataTypeStr=int16  OutDataTypeStr=int16  SaturateOnIntegerOverflow=on
  Add1 : Sum  Inputs=-+  AccumDataTypeStr=int16  OutDataTypeStr=int16  SaturateOnIntegerOverflow=on  LockScale=on
  Compare To Constant : simulink/Logic and Bit Operations/Compare To Constant  relop=<  const=1  OutDataTypeStr=boolean
  Constant Scrambling Sequence : Constant  Value=css  OutDataTypeStr=boolean  SampleTime=tpf
  Constant Valid Signal : Constant  Value=true  OutDataTypeStr=boolean  SampleTime=tpf
  Constant127 : Constant  Value=127  OutDataTypeStr=int16  SampleTime=tpf
  Constant24 : Constant  Value=24  OutDataTypeStr=int16  SampleTime=tpf
  HDL Count Frame Number : hdlsllib/HDL Operations/HDL Counter  CountType=Free running  CountInit=0  CountStep=1  CountMax=25  CountFromType=Initial value  CountFrom=0  CountResetPort=on  CountLoadPort=off  CountEnbPort=off  CountDirPort=off  CountDataType=Unsigned  CountWordLen=16  CountFracLen=0  CountSampTime=1
  Logical OR : Logic  Operator=OR  IconShape=distinctive  AllPortsSameDT=off  OutDataTypeStr=boolean
  Logical XOR : Logic  Operator=XOR  IconShape=distinctive  AllPortsSameDT=off  OutDataTypeStr=boolean
  Resettable Delay : Delay  DelayLength=1  InitialCondition=int16(0)  ExternalReset=Level  SampleTime=tpf
      settings: InputPortMap=u0,r5
  Selector : Selector  IndexMode=Zero-based  InputPortWidth=254  IndexOptions=Starting index (port)  Indices=[1 3]  OutputSizes=24
  Switch : Switch  Threshold=127
  Switch1 : Switch  Criteria=u2 ~= 0
  s1b : Outport
  f1v : Outport  Port=2
  wires:
  s0b/1 -> Switch1/1, Logical XOR/1
  frs/1 -> HDL Count Frame Number/1, Logical OR/1
  HDL Count Frame Number/1 -> Compare To Constant/1
  Compare To Constant/1 -> Switch1/2, Logical OR/2
  Resettable Delay/1 -> Add/2, Selector/2
  Constant Scrambling Sequence/1 -> Selector/1
  Selector/1 -> Logical XOR/2
  Constant Valid Signal/1 -> f1v/1
  Constant24/1 -> Add/1
  Switch/1 -> Resettable Delay/1
  Add/1 -> Add1/2, Switch/2, Switch/3
  Add1/1 -> Switch/1
  Constant127/1 -> Add1/1
  Logical OR/1 -> Resettable Delay/2
  Logical XOR/1 -> Switch1/3
  Switch1/1 -> s1b/1

== system tx80211a5s/dut_pl5s/PL_dut/BPSK Modulate/BPSK Modulate Baseband ==
  bits : Inport
  Constant0 : Constant  Value=0  OutDataTypeStr=fixdt(1,16,14)  SampleTime=tps
  Constant1 : Constant  OutDataTypeStr=int8  SampleTime=tps
  Constant2 : Constant  Value=2  OutDataTypeStr=int8  SampleTime=tps
  Data Type Conversion : DataTypeConversion  OutDataTypeStr=int8
  Data Type Conversion1 : DataTypeConversion  OutDataTypeStr=fixdt(1,16,14)  SaturateOnIntegerOverflow=on
      settings: AttributesFormatString=%<OutDataTypeStr>
  Product : Product  OutDataTypeStr=int8  SaturateOnIntegerOverflow=on
  Real-Imag to Complex : RealImagToComplex
  Subtract : Sum  Inputs=+-  OutDataTypeStr=int8  SaturateOnIntegerOverflow=on
  symbols : Outport
  wires:
  bits/1 -> Data Type Conversion/1
  Data Type Conversion/1 -> Product/1
  Constant2/1 -> Product/2
  Constant1/1 -> Subtract/2
  Product/1 -> Subtract/1
  Subtract/1 -> Data Type Conversion1/1
  Data Type Conversion1/1 -> Real-Imag to Complex/1
  Real-Imag to Complex/1 -> symbols/1
  Constant0/1 -> Real-Imag to Complex/2

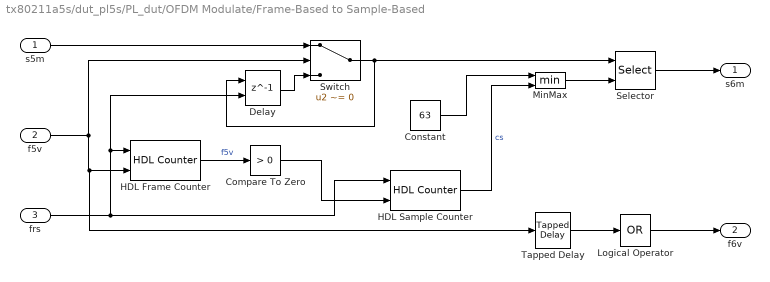
== system tx80211a5s/dut_pl5s/PL_dut/OFDM Modulate/Frame-Based to Sample-Based ==
  s5m : Inport
  f5v : Inport  Port=2
  frs : Inport  Port=3
  Compare To Zero : simulink/Logic and Bit Operations/Compare To Zero  relop=>  OutDataTypeStr=boolean
  Constant : Constant  Value=63  OutDataTypeStr=uint8  SampleTime=tps
  Delay : Delay  DelayLength=1  ExternalReset=Level  SampleTime=tps
      settings: InputPortMap=u0,r5
  HDL Frame Counter : hdlsllib/HDL Operations/HDL Counter  CountType=Free running  CountInit=0  CountStep=1  CountMax=25  CountFromType=Initial value  CountFrom=0  CountResetPort=on  CountLoadPort=off  CountEnbPort=on  CountDirPort=off  CountDataType=Unsigned  CountWordLen=8  CountFracLen=0  CountSampTime=1
  HDL Sample Counter : hdlsllib/HDL Operations/HDL Counter  CountType=Count limited  CountInit=0  CountStep=1  CountMax=nspf-1  CountFromType=Initial value  CountFrom=0  CountResetPort=on  CountLoadPort=off  CountEnbPort=on  CountDirPort=off  CountDataType=Unsigned  CountWordLen=8  CountFracLen=0  CountSampTime=1
  Logical Operator : Logic  Operator=OR  Inputs=1  AllPortsSameDT=off  OutDataTypeStr=boolean
  MinMax : MinMax  Inputs=2
  Selector : Selector  IndexMode=Zero-based  InputPortWidth=64  IndexOptions=Starting index (port)  Indices=[1 3]  OutputSizes=1
  Switch : Switch  Criteria=u2 ~= 0
  Tapped Delay : simulink/Discrete/Tapped Delay  vinit=0  samptime=tps  NumDelays=64  DelayOrder=Oldest  includeCurrent=off
  s6m : Outport
  f6v : Outport  Port=2
  wires:
  s5m/1 -> Switch/1
  f5v/1 -> Tapped Delay/1, HDL Frame Counter/2, Switch/2
  Delay/1 -> Switch/3
  frs/1 -> HDL Frame Counter/1, Delay/2, HDL Sample Counter/1
  Switch/1 -> Delay/1, Selector/1
  Selector/1 -> s6m/1
  Compare To Zero/1 -> HDL Sample Counter/2
  HDL Sample Counter/1 -> MinMax/2  "cs"
  Constant/1 -> MinMax/1
  MinMax/1 -> Selector/2
  HDL Frame Counter/1 -> Compare To Zero/1  "f5v"
  Tapped Delay/1 -> Logical Operator/1
  Logical Operator/1 -> f6v/1
